simulink model "Sim19"  (R2019a)
settings: Solver=VariableStepAuto  StartTime=0.0  StopTime=10.0  RelTol=1e-3
settings Model: Creator=fbleo  LastModifiedBy=fbleo

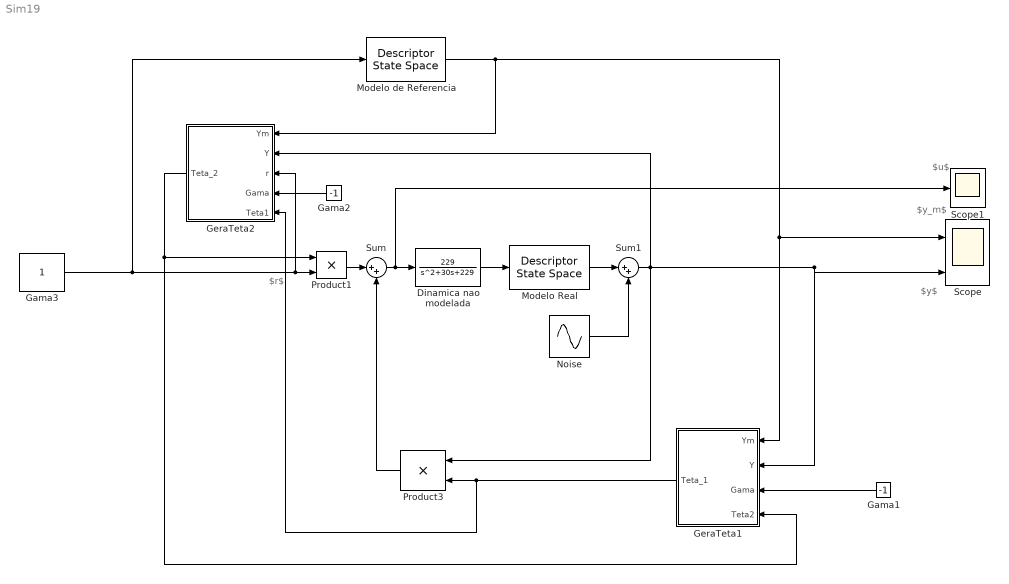
== system Sim19 ==
  note: $y_m$
  note: $u$
  note: $y$
  note: $r$
  Dinamica nao modelada : TransferFcn  Numerator=[229]  Denominator=[1 30 229]
  Gama1 : Constant  Value=-1
  Gama2 : Constant  Value=-1
  Gama3 : Constant
  GeraTeta1 : Subsystem
  GeraTeta2 : Subsystem
  Modelo Real : DescriptorStateSpace  A=-1  B=2  D=0  InitialCondition=0.5
  Modelo de Referencia : DescriptorStateSpace  A=-3  B=3  D=0  InitialCondition=0
  Noise : Sin  Amplitude=0.1  Frequency=16.1  SampleTime=0
  Product1 : Product
  Product3 : Product
  Scope : Scope  NumInputPorts=2
  Scope1 : Scope
  Sum : Sum  Inputs=|++
  Sum1 : Sum  Inputs=|++
  wires:
  Gama1/1 -> GeraTeta1/3(Gama)
  Gama3/1 -> Product1/2, GeraTeta2/3(r), Modelo de Referencia/1
  Modelo de Referencia/1 -> GeraTeta2/1(Ym), GeraTeta1/1(Ym), Scope/1
  Sum1/1 -> GeraTeta2/2(Y), GeraTeta1/2(Y), Scope/2, Product3/1
  Product1/1 -> Sum/1
  Noise/1 -> Sum1/2
  Modelo Real/1 -> Sum1/1
  Dinamica nao modelada/1 -> Modelo Real/1
  Sum/1 -> Scope1/1, Dinamica nao modelada/1
  Product3/1 -> Sum/2
  Gama2/1 -> GeraTeta2/4(Gama)
  GeraTeta1/1(Teta_1) -> GeraTeta2/5(Teta1), Product3/2
  GeraTeta2/1(Teta_2) -> GeraTeta1/4("Teta2 "), Product1/1

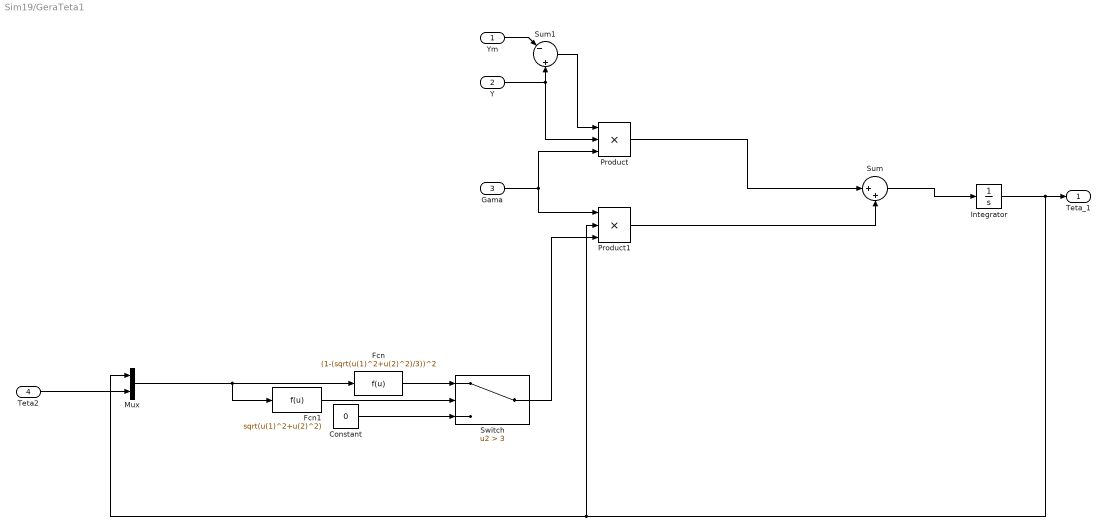
== system Sim19/GeraTeta1 ==
  Ym : Inport
  Y : Inport  Port=2
  Gama : Inport  Port=3
  "Teta2 " : Inport  Port=4
  Constant : Constant  Value=0
  Fcn : Fcn  Expr=(1-(sqrt(u(1)^2+u(2)^2)/3))^2
  Fcn1 : Fcn  Expr=sqrt(u(1)^2+u(2)^2)
  Integrator : Integrator  InitialCondition=-0.65
  Mux : Mux  Inputs=2
  Product : Product  Inputs=3
  Product1 : Product  Inputs=3
  Sum : Sum  Inputs=|++
  Sum1 : Sum  Inputs=|-||+
  Switch : Switch  Criteria=u2 > Threshold  Threshold=3
  Teta_1 : Outport
  wires:
  Ym/1 -> Sum1/1
  Sum1/1 -> Product/1
  Y/1 -> Sum1/2, Product/2
  Gama/1 -> Product1/1, Product/3
  Product/1 -> Sum/1
  Sum/1 -> Integrator/1
  Integrator/1 -> Mux/1, Product1/2, Teta_1/1
  "Teta2 "/1 -> Mux/2
  Switch/1 -> Product1/3
  Product1/1 -> Sum/2
  Fcn/1 -> Switch/1
  Mux/1 -> Fcn1/1, Fcn/1
  Constant/1 -> Switch/3
  Fcn1/1 -> Switch/2

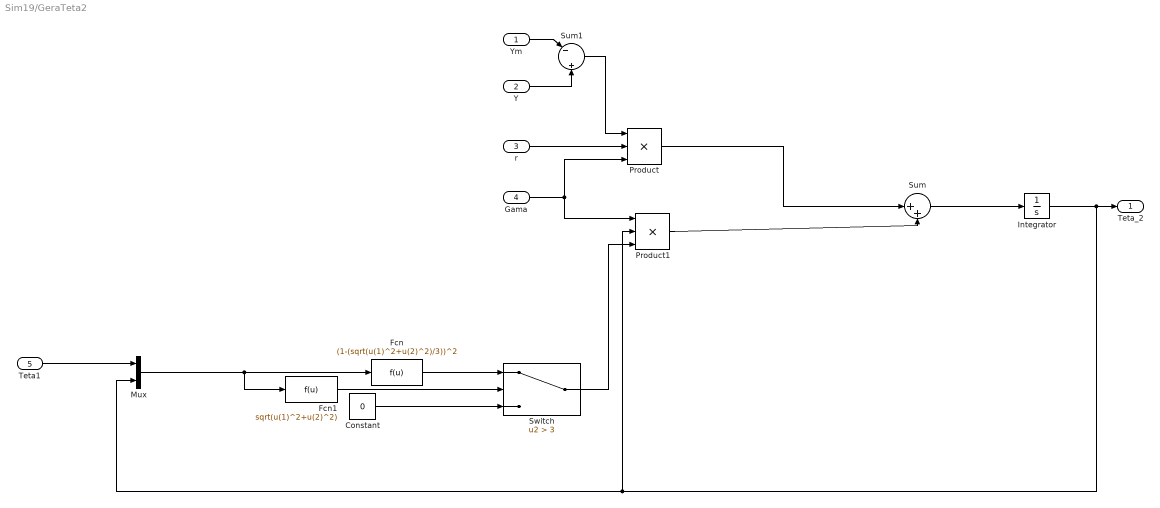
== system Sim19/GeraTeta2 ==
  Ym : Inport
  Y : Inport  Port=2
  r : Inport  Port=3
  Gama : Inport  Port=4
  Teta1 : Inport  Port=5
  Constant : Constant  Value=0
  Fcn : Fcn  Expr=(1-(sqrt(u(1)^2+u(2)^2)/3))^2
  Fcn1 : Fcn  Expr=sqrt(u(1)^2+u(2)^2)
  Integrator : Integrator  InitialCondition=1.14
  Mux : Mux  Inputs=2
  Product : Product  Inputs=3
  Product1 : Product  Inputs=3
  Sum : Sum  Inputs=|++
  Sum1 : Sum  Inputs=|-||+
  Switch : Switch  Criteria=u2 > Threshold  Threshold=3
  Teta_2 : Outport
  wires:
  Ym/1 -> Sum1/1
  Y/1 -> Sum1/2
  Sum1/1 -> Product/1
  r/1 -> Product/2
  Gama/1 -> Product1/1, Product/3
  Product/1 -> Sum/1
  Sum/1 -> Integrator/1
  Integrator/1 -> Mux/2, Product1/2, Teta_2/1
  Product1/1 -> Sum/2
  Mux/1 -> Fcn1/1, Fcn/1
  Fcn1/1 -> Switch/2
  Constant/1 -> Switch/3
  Switch/1 -> Product1/3
  Fcn/1 -> Switch/1
  Teta1/1 -> Mux/1
